simulink model "SVPWM_V1"  (R2023a)
settings: Solver=FixedStepDiscrete  StartTime=0.0  StopTime=1  FixedStep=1/100000  RelTol=1e-3
PreLoadFcn:
  | run("Data.m")
values from neighbouring files (symbols this model uses):
  LdTrq = -10    [Data.m]
  Ts = 1/10000    (= 0.0001)    [Data.m]
  Udc = 38    [Data.m]
libraries: simulink x9, mcbcontrolslib x2, autolibpmsmexterior x1
CloseFcn:
  | clear
settings Model: Creator=25313  LastModifiedBy=25313
settings OptimizationCC: DefaultParameterBehavior=Inlined  EnhancedBackFolding=on  PassReuseOutputArgsAs=Individual arguments  ZeroExternalMemoryAtStartup=off  ZeroInternalMemoryAtStartup=off  OptimizeBlockOrder=speed  DifferentSizesBufferReuse=on  OptimizationCustomize=off  EfficientTunableParamExpr=on
settings DebuggingCC: ParameterOverflowMsg=none  ParameterUnderflowMsg=error  ParameterPrecisionLossMsg=none  ParameterTunabilityLossMsg=error
settings SFSimCC: MATLABDynamicMemAlloc=off
settings RTWCC: Description=Embedded Coder  SystemTargetFile=ert.tlc  TemplateMakefile=ert_default_tmf
settings CodeAppCC: ForceParamTrailComments=on  IgnoreCustomStorageClasses=off  OperatorAnnotations=on  SimulinkDataObjDesc=on  SFDataObjDesc=on  InsertBlockDesc=on
settings ERTTargetCC: TargetLangStandard=C99 (ISO)  GenerateSampleERTMain=on  InlinedParameterPlacement=NonHierarchical  ERTCustomFileTemplate=example_file_process.tlc

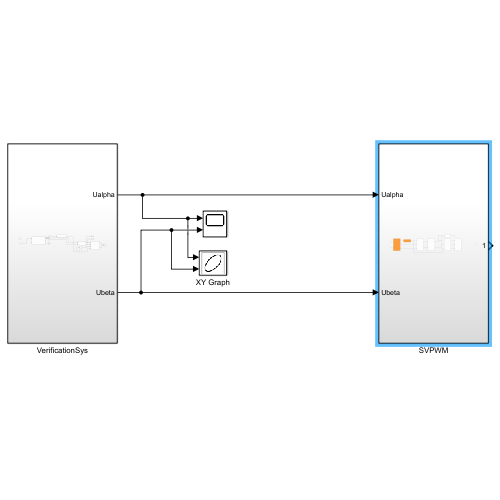
[thumbnail: Simulink's stored preview of the top-level diagram]
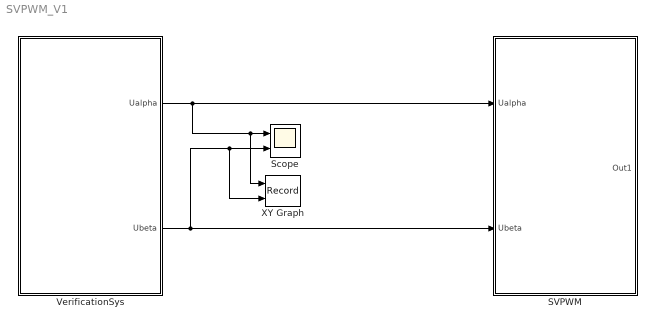
== system SVPWM_V1 ==
  SVPWM : Subsystem
  Scope : Scope  NumInputPorts=2
  VerificationSys : Subsystem
  XY Graph : Record  FileSettingsInternal="{\"entries\":[{\"content\":{\"excelSettings\":{\"content\":{},\"type\":\"Streamout.ExcelSettings\"}},\"type\":\"Streamout.FileSettingStorage\",\"uuid\":\"\"}],\"packageUris\":[\"http:\\/\\/schema.mathworks.com\\/mf0\\/streamout_blocks\\/R2020a\"],\"version\":\"1.0\"}"  Layout=[1 1]  SignalsInternal="{\"entries\":[{\"content\":{\"signals\":[{\"content\":{\"blockPath\":[],\"dimensions\":[1],\"domain\":\"\",\"lineColor\":\"#a2142f\",\"plots\":[1],\"port\":1,\"sid\":[\"\"],\"signalID\":1546,\"signalName\":\"VerificationSys:1\"},\"type\":\"RecordBlkView.Signal\",\"uuid\":\"\"},{\"content\":{\"blockPath\":[],\"dimensions\":[1],\"domain\":\"\",\"lineColor\":\"#139fff\",\"plots\":[1],\"port\":2,\"sid\":[\"\"],\"signalID\":1550,\"signalName\":\"VerificationSys:2\"},\"type\":\"RecordBlkView.Signal\",\"uuid\":\"\"}]},\"type\":\"RecordBlkView.InputSignals\",\"uuid\":\"\"}],\"packageUris\":[\"http:\\/\\/schema.mathworks.com\\/mf0\\/streamout_blocks\\/R2020a\"],\"version\":\"1.0\"}"  VisualizationBindings="{\"xyplotplugin\":{\"info\":[{\"series\":[{\"bindingParametersList\":[{\"parameter\":\"X-Axis\",\"signalID\":1546,\"signalName\":\"VerificationSys:1\"},{\"parameter\":\"Y-Axis\",\"signalID\":1550,\"signalName\":\"VerificationSys:2\"}],\"seriesID\":14155}],\"subplotID\":1}]}}"  CompatibilityTag=XY
  wires:
  VerificationSys/1(Ualpha) -> XY Graph/1, Scope/1, SVPWM/1(Ualpha)
  VerificationSys/2(Ubeta) -> SVPWM/2(Ubeta), XY Graph/2, Scope/2

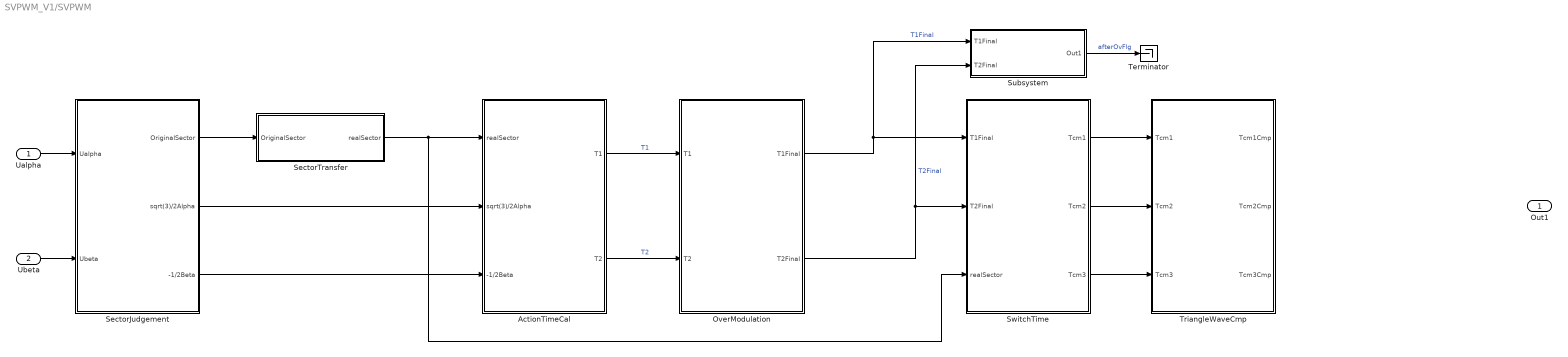
== system SVPWM_V1/SVPWM ==
  Ualpha : Inport
  Ubeta : Inport  Port=2
  ActionTimeCal : Subsystem
  OverModulation : Subsystem
  SectorJudgement : Subsystem
  SectorTransfer : Subsystem
  Subsystem : Subsystem
  SwitchTime : Subsystem
  Terminator : Terminator
  TriangleWaveCmp : Subsystem
  Out1 : Outport
  wires:
  Ualpha/1 -> SectorJudgement/1(Ualpha)
  Ubeta/1 -> SectorJudgement/2(Ubeta)
  SectorJudgement/1(OriginalSector) -> SectorTransfer/1(OriginalSector)
  SectorTransfer/1(realSector) -> SwitchTime/3(realSector), ActionTimeCal/1(realSector)
  SectorJudgement/2(sqrt(3)/2Alpha) -> ActionTimeCal/2(sqrt(3)/2Alpha)
  SectorJudgement/3(-1/2Beta) -> ActionTimeCal/3(-1/2Beta)
  ActionTimeCal/1(T1) -> OverModulation/1(T1)  "T1"
  ActionTimeCal/2(T2) -> OverModulation/2(T2)  "T2"
  OverModulation/1(T1Final) -> Subsystem/1(T1Final), SwitchTime/1(T1Final)  "T1Final"
  OverModulation/2(T2Final) -> Subsystem/2(T2Final), SwitchTime/2(T2Final)  "T2Final"
  Subsystem/1(Out1) -> Terminator/1  "afterOvFlg"
  SwitchTime/1(Tcm1) -> TriangleWaveCmp/1(Tcm1)
  SwitchTime/2(Tcm2) -> TriangleWaveCmp/2(Tcm2)
  SwitchTime/3(Tcm3) -> TriangleWaveCmp/3(Tcm3)

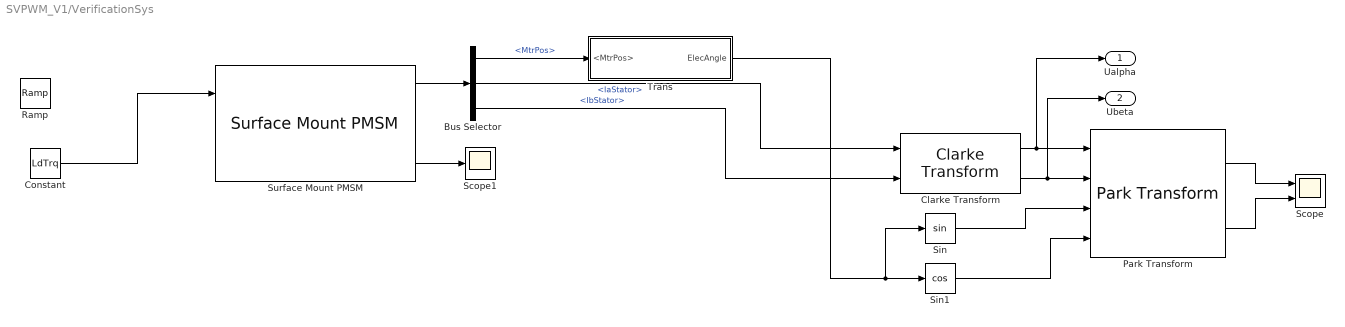
== system SVPWM_V1/VerificationSys ==
  Bus Selector : BusSelector  OutputSignals=MtrPos,IaStator,IbStator
  Clarke Transform : mcbcontrolslib/Clarke Transform  VariantControl=Variant2
      settings: LibrarySourceBlock=mcbhdllib/Controls/Math Transforms/Clarke Transform
  Constant : Constant  Value=LdTrq
  Park Transform : mcbcontrolslib/Park Transform  AxisAlignment=D-axis
      settings: LibrarySourceBlock=mcbhdllib/Controls/Math Transforms/Park Transform
  Ramp : simulink/Sources/Ramp  slope=-10  start=0  InitialOutput=0
  Scope : Scope  NumInputPorts=2
  Scope1 : Scope
  Sin : Trigonometry
  Sin1 : Trigonometry  Operator=cos
  Surface Mount PMSM : autolibpmsmexterior/Surface Mount PMSM  port_config=Torque  sim_type=Discrete  Ts=1/10000  FilePath=E:\Sandbox\Bauto\Work\surfacepmsm_motordata.m  P=4  Rs=.2  Ldq_=3.752e-4  KConstText=Permanent flux linkage constant (lambda_pm):  lambda_pm=0.1194  Ke=159.9771  Kt=1.323  mechanical=[0.0027, 4.924e-4, 0]  idq0=[0 0]  theta_init=0  omega_init=0  KConst=0.1194  lambda_pm_calc=0.1194  RefBlkName='autolibpmsmexterior/Surface Mount PMSM'  aMode=1  Ldq="[0.0003752   0.0003752]"
      settings: LibrarySourceBlock=autolibemachines/Surface Mount PMSM
  Trans : Subsystem
  Ualpha : Outport
  Ubeta : Outport  Port=2
  wires:
  Surface Mount PMSM/1 -> Bus Selector/1
  Constant/1 -> Surface Mount PMSM/1
  Clarke Transform/2 -> Ubeta/1, Park Transform/2
  Bus Selector/2 -> Clarke Transform/1  "<IaStator>"
  Bus Selector/3 -> Clarke Transform/2  "<IbStator>"
  Bus Selector/1 -> Trans/1(<MtrPos>)  "<MtrPos>"
  Trans/1(ElecAngle) -> Sin/1, Sin1/1
  Sin/1 -> Park Transform/3
  Sin1/1 -> Park Transform/4
  Park Transform/1 -> Scope/1
  Park Transform/2 -> Scope/2
  Clarke Transform/1 -> Ualpha/1, Park Transform/1
  Surface Mount PMSM/3 -> Scope1/1

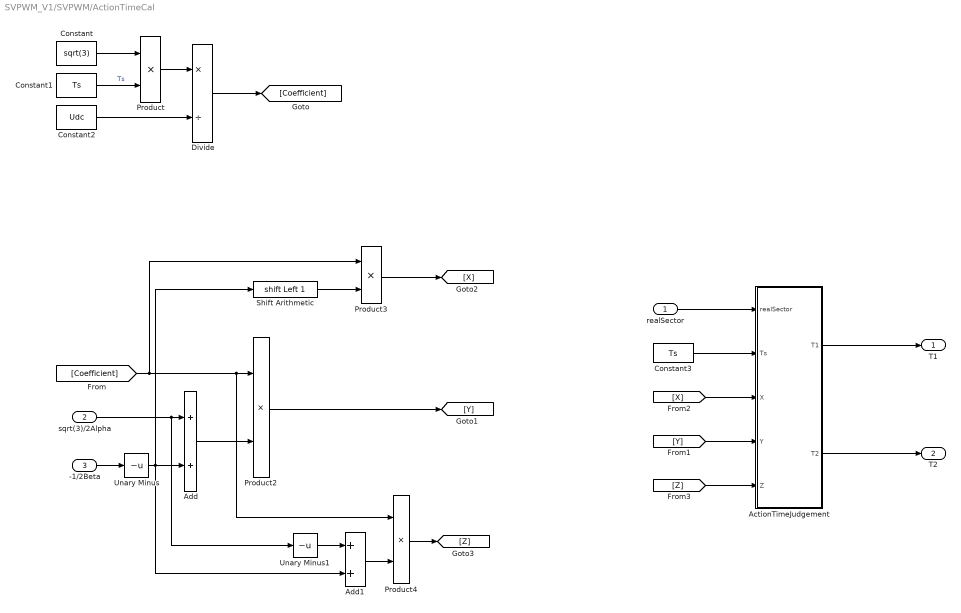
== system SVPWM_V1/SVPWM/ActionTimeCal ==
  realSector : Inport
  sqrt(3)/2Alpha : Inport  Port=2
  -1/2Beta : Inport  Port=3
  ActionTimeJudgement : MATLAB Function  TreatAsAtomicUnit=on
  Add : Sum
  Add1 : Sum
  Constant : Constant  Value=sqrt(3)
  Constant1 : Constant  Value=Ts
  Constant2 : Constant  Value=Udc
  Constant3 : Constant  Value=Ts
  Divide : Product  Inputs=*/
  Product{,2..4} (4 alike) : Product
  Shift Arithmetic : ArithShift  BitShiftNumber=1  BitShiftDirection=Left
  Unary Minus : UnaryMinus
  Unary Minus1 : UnaryMinus
  T1 : Outport
  T2 : Outport  Port=2
  wires:
  Constant/1 -> Product/1
  Constant1/1 -> Product/2  "Ts"
  Product/1 -> Divide/1
  Divide/1 -> [Coefficient]
  [Coefficient] -> Product3/1, Product4/1, Product2/1
  sqrt(3)/2Alpha/1 -> Unary Minus1/1, Add/1
  -1/2Beta/1 -> Unary Minus/1
  Unary Minus/1 -> Add1/2, Add/2, Shift Arithmetic/1
  Add/1 -> Product2/2
  Product2/1 -> [Y]
  Shift Arithmetic/1 -> Product3/2
  Product3/1 -> [X]
  Unary Minus1/1 -> Add1/1
  Add1/1 -> Product4/2
  Product4/1 -> [Z]
  [X] -> ActionTimeJudgement/3(X)
  [Y] -> ActionTimeJudgement/4(Y)
  [Z] -> ActionTimeJudgement/5(Z)
  realSector/1 -> ActionTimeJudgement/1(realSector)
  ActionTimeJudgement/1(T1) -> T1/1
  ActionTimeJudgement/2(T2) -> T2/1
  Constant3/1 -> ActionTimeJudgement/2(Ts)
  Constant2/1 -> Divide/2

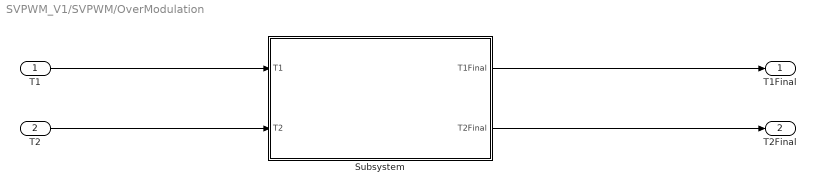
== system SVPWM_V1/SVPWM/OverModulation ==
  T1 : Inport
  T2 : Inport  Port=2
  Subsystem : Subsystem  Variant=on  VariantControl=Choice
  T1Final : Outport
  T2Final : Outport  Port=2
  wires:
  T1/1 -> Subsystem/1(T1)
  T2/1 -> Subsystem/2(T2)
  Subsystem/1(T1Final) -> T1Final/1
  Subsystem/2(T2Final) -> T2Final/1

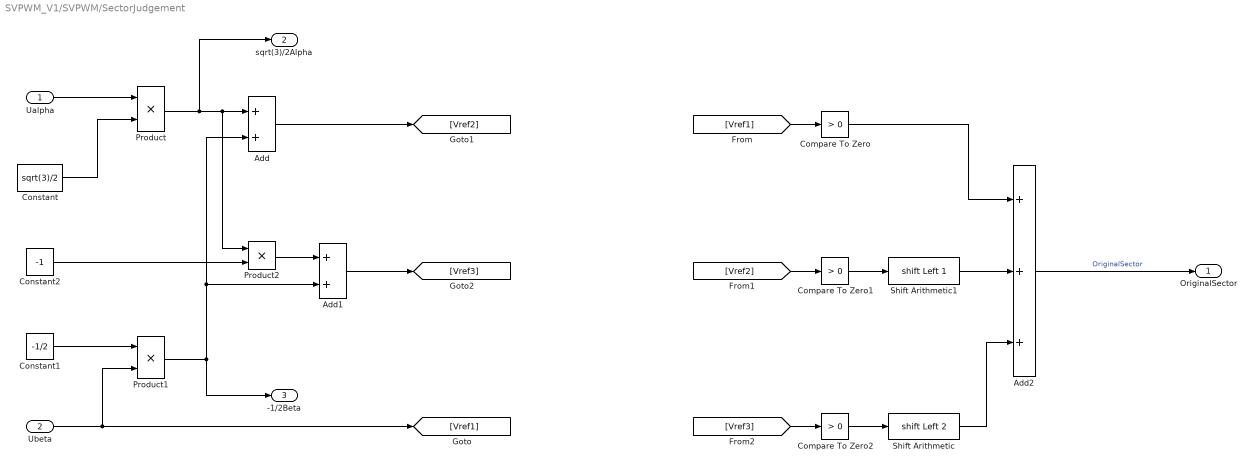
== system SVPWM_V1/SVPWM/SectorJudgement ==
  Ualpha : Inport
  Ubeta : Inport  Port=2
  Add : Sum
  Add1 : Sum
  Add2 : Sum  Inputs=3
  Compare To Zero : simulink/Logic and Bit Operations/Compare To Zero  relop=>  OutDataTypeStr=uint8
  Compare To Zero1 : simulink/Logic and Bit Operations/Compare To Zero  relop=>  OutDataTypeStr=uint8
  Compare To Zero2 : simulink/Logic and Bit Operations/Compare To Zero  relop=>  OutDataTypeStr=uint8
  Constant : Constant  Value=sqrt(3)/2
  Constant1 : Constant  Value=-1/2
  Constant2 : Constant  Value=-1
  Product : Product
  Product1 : Product
  Product2 : Product
  Shift Arithmetic : ArithShift  BitShiftNumber=2  BitShiftDirection=Left
  Shift Arithmetic1 : ArithShift  BitShiftNumber=1  BitShiftDirection=Left
  OriginalSector : Outport
  sqrt(3)/2Alpha : Outport  Port=2
  -1/2Beta : Outport  Port=3
  wires:
  Ubeta/1 -> Product1/2, [Vref1]
  Ualpha/1 -> Product/1
  Constant/1 -> Product/2
  Constant1/1 -> Product1/1
  Product/1 -> sqrt(3)/2Alpha/1, Product2/1, Add/1
  Product1/1 -> -1/2Beta/1, Add1/2, Add/2
  Add/1 -> [Vref2]
  Constant2/1 -> Product2/2
  Product2/1 -> Add1/1
  Add1/1 -> [Vref3]
  [Vref3] -> Compare To Zero2/1
  [Vref2] -> Compare To Zero1/1
  Shift Arithmetic1/1 -> Add2/2
  Shift Arithmetic/1 -> Add2/3
  [Vref1] -> Compare To Zero/1
  Add2/1 -> OriginalSector/1  "OriginalSector"
  Compare To Zero/1 -> Add2/1
  Compare To Zero1/1 -> Shift Arithmetic1/1
  Compare To Zero2/1 -> Shift Arithmetic/1

== system SVPWM_V1/SVPWM/SectorTransfer ==
  note: 3 1 5 4 6 2
      | 1 2 3 4 5 6
  OriginalSector : Inport
  Constant : Constant  Value=[0 2 6 1 4 3 5]
  Selector : Selector  IndexMode=Zero-based  InputPortWidth=7  IndexOptions=Index vector (port)  Indices=[1 3]  OutputSizes=1
  To Workspace : ToWorkspace  VariableName=realSector  SaveFormat=Timeseries  SampleTime=-1
  realSector : Outport
  wires:
  OriginalSector/1 -> Selector/2
  Constant/1 -> Selector/1
  Selector/1 -> To Workspace/1, realSector/1  "realSector"

== system SVPWM_V1/SVPWM/Subsystem ==
  T1Final : Inport
  T2Final : Inport  Port=2
  Add : Sum
  Compare To Constant : simulink/Logic and Bit Operations/Compare To Constant  relop=>  const=Ts  OutDataTypeStr=boolean
  Out1 : Outport
  wires:
  T1Final/1 -> Add/1
  T2Final/1 -> Add/2
  Add/1 -> Compare To Constant/1  "FinalSum"
  Compare To Constant/1 -> Out1/1

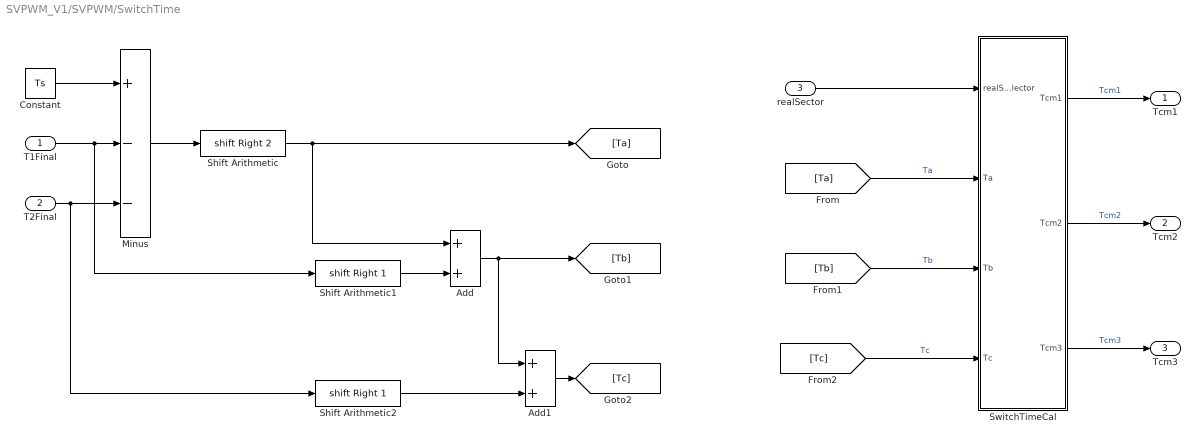
== system SVPWM_V1/SVPWM/SwitchTime ==
  T1Final : Inport
  T2Final : Inport  Port=2
  realSector : Inport  Port=3
  Add : Sum
  Add1 : Sum
  Constant : Constant  Value=Ts
  Minus : Sum  Inputs=+--
  Shift Arithmetic : ArithShift  BitShiftNumber=2  BitShiftDirection=Right
  Shift Arithmetic1 : ArithShift  BitShiftNumber=1  BitShiftDirection=Right
  Shift Arithmetic2 : ArithShift  BitShiftNumber=1  BitShiftDirection=Right
  SwitchTimeCal : MATLAB Function  TreatAsAtomicUnit=on
  Tcm1 : Outport
  Tcm2 : Outport  Port=2
  Tcm3 : Outport  Port=3
  wires:
  T1Final/1 -> Shift Arithmetic1/1, Minus/2
  Constant/1 -> Minus/1
  Minus/1 -> Shift Arithmetic/1
  Shift Arithmetic/1 -> Add/1, [Ta]
  Shift Arithmetic1/1 -> Add/2
  Shift Arithmetic2/1 -> Add1/2
  Add/1 -> [Tb], Add1/1
  T2Final/1 -> Shift Arithmetic2/1, Minus/3
  Add1/1 -> [Tc]
  realSector/1 -> SwitchTimeCal/1(realSelector)
  [Ta] -> SwitchTimeCal/2(Ta)  "Ta"
  [Tb] -> SwitchTimeCal/3(Tb)  "Tb"
  [Tc] -> SwitchTimeCal/4(Tc)  "Tc"
  SwitchTimeCal/1(Tcm1) -> Tcm1/1  "Tcm1"
  SwitchTimeCal/2(Tcm2) -> Tcm2/1  "Tcm2"
  SwitchTimeCal/3(Tcm3) -> Tcm3/1  "Tcm3"

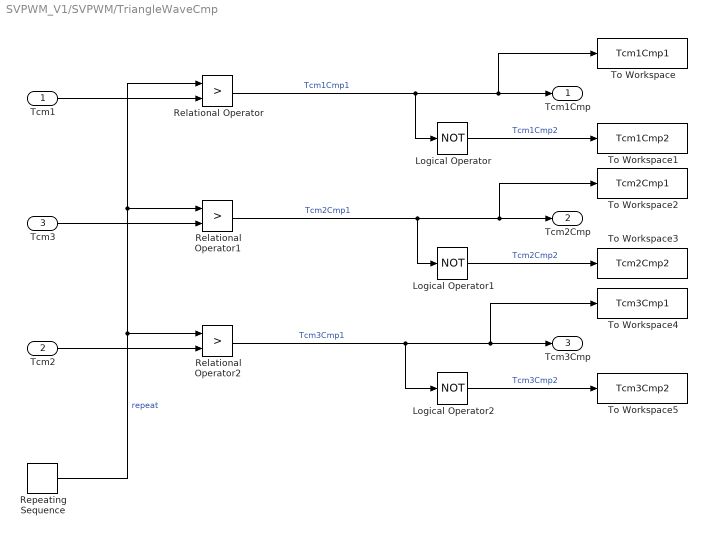
== system SVPWM_V1/SVPWM/TriangleWaveCmp ==
  Tcm1 : Inport
  Tcm2 : Inport  Port=2
  Tcm3 : Inport  Port=3
  Logical Operator : Logic  Operator=NOT  AllPortsSameDT=off  OutDataTypeStr=boolean
  Logical Operator1 : Logic  Operator=NOT  AllPortsSameDT=off  OutDataTypeStr=boolean
  Logical Operator2 : Logic  Operator=NOT  AllPortsSameDT=off  OutDataTypeStr=boolean
  Relational Operator : RelationalOperator  Operator=>  OutDataTypeStr=boolean  RndMeth=Simplest  InputSameDT=off
  Relational Operator1 : RelationalOperator  Operator=>  OutDataTypeStr=boolean  RndMeth=Simplest  InputSameDT=off
  Relational Operator2 : RelationalOperator  Operator=>  OutDataTypeStr=boolean  RndMeth=Simplest  InputSameDT=off
  Repeating Sequence : simulink/Sources/Repeating Sequence  rep_seq_t=[0 Ts/2 Ts]  rep_seq_y=[0 Ts/2 0]
  To Workspace : ToWorkspace  VariableName=Tcm1Cmp1  SaveFormat=Timeseries  SampleTime=-1
  To Workspace1 : ToWorkspace  VariableName=Tcm1Cmp2  SaveFormat=Timeseries  SampleTime=-1
  To Workspace2 : ToWorkspace  VariableName=Tcm2Cmp1  SaveFormat=Timeseries  SampleTime=-1
  To Workspace3 : ToWorkspace  VariableName=Tcm2Cmp2  SaveFormat=Timeseries  SampleTime=-1
  To Workspace4 : ToWorkspace  VariableName=Tcm3Cmp1  SaveFormat=Timeseries  SampleTime=-1
  To Workspace5 : ToWorkspace  VariableName=Tcm3Cmp2  SaveFormat=Timeseries  SampleTime=-1
  Tcm1Cmp : Outport
  Tcm2Cmp : Outport  Port=2
  Tcm3Cmp : Outport  Port=3
  wires:
  Repeating Sequence/1 -> Relational Operator1/1, Relational Operator/1, Relational Operator2/1  "repeat"
  Tcm1/1 -> Relational Operator/2
  Relational Operator/1 -> Logical Operator/1, To Workspace/1, Tcm1Cmp/1  "Tcm1Cmp1"
  Tcm3/1 -> Relational Operator1/2
  Tcm2/1 -> Relational Operator2/2
  Relational Operator1/1 -> Logical Operator1/1, To Workspace2/1, Tcm2Cmp/1  "Tcm2Cmp1"
  Relational Operator2/1 -> Logical Operator2/1, To Workspace4/1, Tcm3Cmp/1  "Tcm3Cmp1"
  Logical Operator/1 -> To Workspace1/1  "Tcm1Cmp2"
  Logical Operator1/1 -> To Workspace3/1  "Tcm2Cmp2"
  Logical Operator2/1 -> To Workspace5/1  "Tcm3Cmp2"

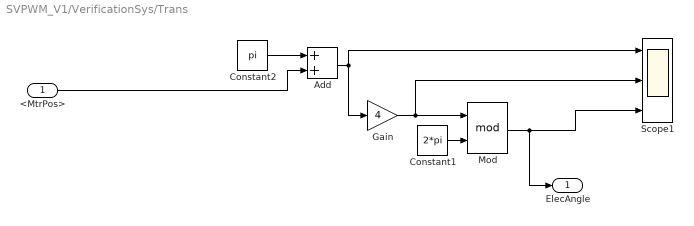
== system SVPWM_V1/VerificationSys/Trans ==
  <MtrPos> : Inport
  Add : Sum
  Constant1 : Constant  Value=2*pi
  Constant2 : Constant  Value=pi
  Gain : Gain  Gain=4
  Mod : Math  Operator=mod
  Scope1 : Scope  NumInputPorts=3
  ElecAngle : Outport
  wires:
  Constant2/1 -> Add/1
  Gain/1 -> Scope1/2, Mod/1
  <MtrPos>/1 -> Add/2
  Constant1/1 -> Mod/2
  Mod/1 -> ElecAngle/1, Scope1/3
  Add/1 -> Gain/1, Scope1/1

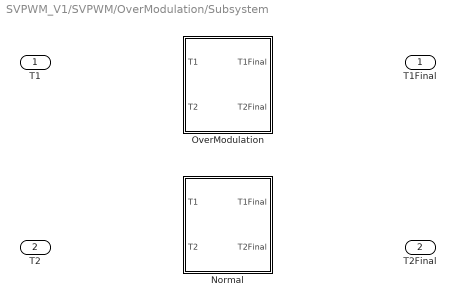
== system SVPWM_V1/SVPWM/OverModulation/Subsystem ==
  T1 : Inport
  T2 : Inport  Port=2
  Normal : Subsystem  VariantControl=OverModulationOnOFF == 0
  OverModulation : Subsystem  VariantControl=OverModulationOnOFF == 1
  T1Final : Outport
  T2Final : Outport  Port=2

== system SVPWM_V1/SVPWM/OverModulation/Subsystem/Normal ==
  T1 : Inport
  T2 : Inport  Port=2
  T1Final : Outport
  T2Final : Outport  Port=2
  wires:
  T2/1 -> T2Final/1
  T1/1 -> T1Final/1

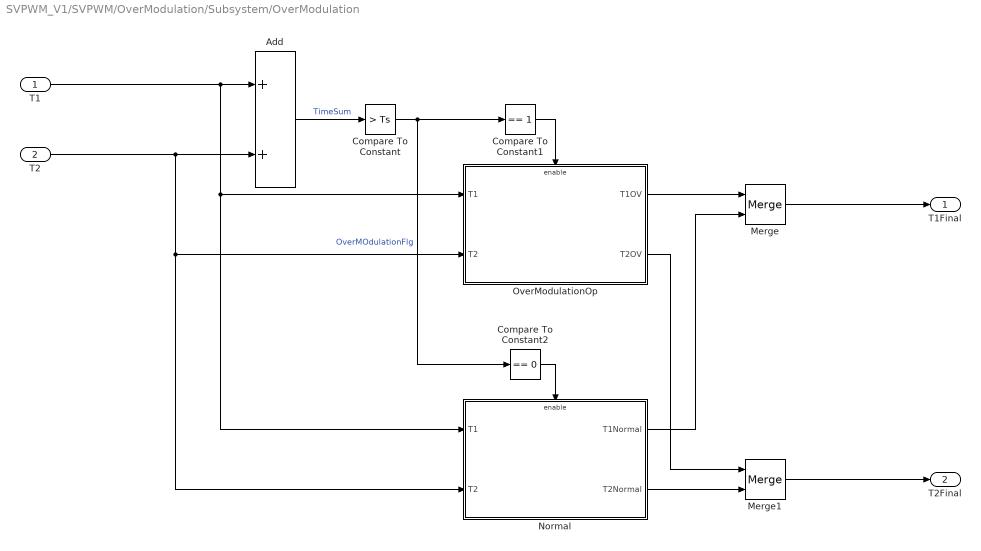
== system SVPWM_V1/SVPWM/OverModulation/Subsystem/OverModulation ==
  T1 : Inport
  T2 : Inport  Port=2
  Add : Sum
  Compare To Constant : simulink/Logic and Bit Operations/Compare To Constant  relop=>  const=Ts  OutDataTypeStr=boolean
  Compare To Constant1 : simulink/Logic and Bit Operations/Compare To Constant  relop===  const=1  OutDataTypeStr=boolean
  Compare To Constant2 : simulink/Logic and Bit Operations/Compare To Constant  relop===  const=0  OutDataTypeStr=boolean
  Merge : Merge
  Merge1 : Merge
  Normal : Subsystem  TreatAsAtomicUnit=on
  OverModulationOp : Subsystem  TreatAsAtomicUnit=on
  T1Final : Outport
  T2Final : Outport  Port=2
  wires:
  Add/1 -> Compare To Constant/1  "TimeSum"
  T1/1 -> Normal/1(T1), OverModulationOp/1(T1), Add/1
  T2/1 -> Normal/2(T2), OverModulationOp/2(T2), Add/2
  Normal/2(T2Normal) -> Merge1/2
  OverModulationOp/2(T2OV) -> Merge1/1
  OverModulationOp/1(T1OV) -> Merge/1
  Compare To Constant/1 -> Compare To Constant2/1, Compare To Constant1/1  "OverMOdulationFlg"
  Compare To Constant1/1 -> OverModulationOp/Enable
  Compare To Constant2/1 -> Normal/Enable
  Normal/1(T1Normal) -> Merge/2
  Merge/1 -> T1Final/1
  Merge1/1 -> T2Final/1

== system SVPWM_V1/SVPWM/OverModulation/Subsystem/OverModulation/Normal ==
  T1 : Inport
  T2 : Inport  Port=2
  Enable : EnablePort
  T1Normal : Outport
  T2Normal : Outport  Port=2
  wires:
  T1/1 -> T1Normal/1  "T1Normal"
  T2/1 -> T2Normal/1  "T2Normal"

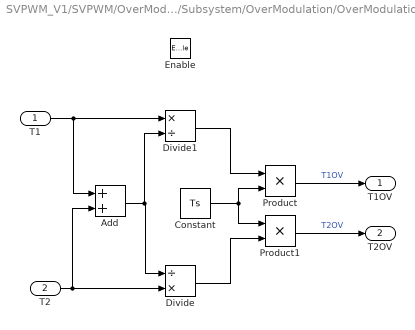
== system SVPWM_V1/SVPWM/OverModulation/Subsystem/OverModulation/OverModulationOp ==
  T1 : Inport
  T2 : Inport  Port=2
  Enable : EnablePort
  Add : Sum
  Constant : Constant  Value=Ts
  Divide : Product  Inputs=/*
  Divide1 : Product  Inputs=*/
  Product : Product
  Product1 : Product
  T1OV : Outport  InitialOutput=0
  T2OV : Outport  Port=2
  wires:
  T1/1 -> Divide1/1, Add/1
  T2/1 -> Divide/2, Add/2
  Add/1 -> Divide1/2, Divide/1
  Constant/1 -> Product1/1, Product/2
  Divide1/1 -> Product/1
  Divide/1 -> Product1/2
  Product/1 -> T1OV/1  "T1OV"
  Product1/1 -> T2OV/1  "T2OV"

== matlab function SVPWM_V1/SVPWM/SwitchTime/SwitchTimeCal ==
  data: realSelector input; Ta input; Tcm1 output; Tb input; Tc input; Tcm2 output; Tcm3 output
function [Tcm1,Tcm2,Tcm3] = TcmCal(realSelector,Ta,Tb,Tc)

tcm1 = 0;
tcm2 = 0;
tcm3 = 0;

if realSelector == 1
    tcm1 = Ta;
    tcm2 = Tb;
    tcm3 = Tc;
elseif realSelector == 2
    tcm1 = Tb;
    tcm2 = Ta;
    tcm3 = Tc;
elseif realSelector == 3
    tcm1 = Tc;
    tcm2 = Ta;
    tcm3 = Tb;
elseif realSelector == 4
    tcm1 = Tc;
    tcm2 = Tb;
    tcm3 = Ta;
elseif realSelector == 5
    tcm1 = Tb;
    tcm2 = Tc;
    tcm3 = Ta;
elseif realSelector == 6
    tcm1 = Ta;
    tcm2 = Tc;
    tcm3 = Tb;

end
Tcm1 = tcm1;
Tcm2 = tcm2;
Tcm3 = tcm3;
end

== matlab function SVPWM_V1/SVPWM/ActionTimeCal/ActionTimeJudgement ==
  data: realSector input; Ts input; X input; T1 output; Y input; Z input; T2 output
function [T1,T2] = judgement(realSector, Ts, X, Y, Z)

t1 = 0;
t2 = 0;
t0 = 0;
t7 = 0;

if realSector == 1

    t1 = -Z;
    t2 = X;


elseif realSector == 2

    t1 = Z;
    t2 = Y;


elseif realSector == 3
    t1 = X;
    t2 = -Y;


elseif realSector == 4

    t1 = -X;
    t2 = Z;


elseif realSector == 5

    t1 = -Y;
    t2 = -Z;


elseif realSector == 6

    t1 = Y;
    t2 = -X;

end


T1 = t1;
T2 = t2;
t0 = (Ts-t1-t2)/2;
t7 = (Ts-t1-t2)/2;

end
